simulink model "FinalSystem_WithRT"  (R2022b)
settings: Solver=FixedStepAuto  StartTime=0.0  StopTime=10.0  FixedStep=1e-3  RelTol=1e-3  EnableMultiTasking=on
undefined symbols (not defined in the file): D0, D1, D10, D11, D12, D13, D2, D3, D4, D5, D6, D7, D8, D9, PTA0, PTA1, PTA2, PTB23, PTB9, PTC16, PTC17, PTC2, PTC3, PTC4, PTD0, PTD1, PTD2, PTD3
libraries: frdmk64flib x17
settings Model: ExtModeTrigDuration=5  Creator=sarahalabdulrazzak  LastModifiedBy=TheCoaler
settings SolverCC: AlgebraicLoopSolver=TrustRegion
settings OptimizationCC: EnhancedBackFolding=on  PassReuseOutputArgsAs=Individual arguments  ZeroExternalMemoryAtStartup=off  ZeroInternalMemoryAtStartup=off  MaxStackSize=64  OptimizeBlockOrder=speed  DifferentSizesBufferReuse=on  OptimizationCustomize=off  EfficientTunableParamExpr=on
settings DebuggingCC: ParameterTunabilityLossMsg=error  UnconnectedInputMsg=warning  UnconnectedOutputMsg=warning  UnconnectedLineMsg=warning  SFMachineParentedDataDiag=warning
settings HardwareCC: ProdBitPerPointer=32  ProdBitPerSizeT=32  ProdBitPerPtrDiffT=32  ProdLargestAtomicInteger=Long  ProdLargestAtomicFloat=Double  ProdWordSize=32  ProdHWDeviceType=ARM Compatible->ARM Cortex
settings ModelReferenceCC: EnableRefExpFcnMdlSchedulingChecks=on
settings SFSimCC: MATLABDynamicMemAlloc=off
settings RTWCC: Description=Embedded Coder  SystemTargetFile=ert.tlc  HardwareBoard=NXP FRDM-K64F  TLCOptions="-aInlineSetEventsForThisBaseRateFcn=TLC_FALSE -aSuppressMultiTaskScheduler=TLC_FALSE  -aRateBasedStepFcn=0"  TemplateMakefile=ert_default_tmf  Toolchain=GNU Tools for ARM Embedded Processors
settings CodeAppCC: ForceParamTrailComments=on  IgnoreCustomStorageClasses=off  OperatorAnnotations=on  SimulinkDataObjDesc=on  SFDataObjDesc=on  InsertBlockDesc=on

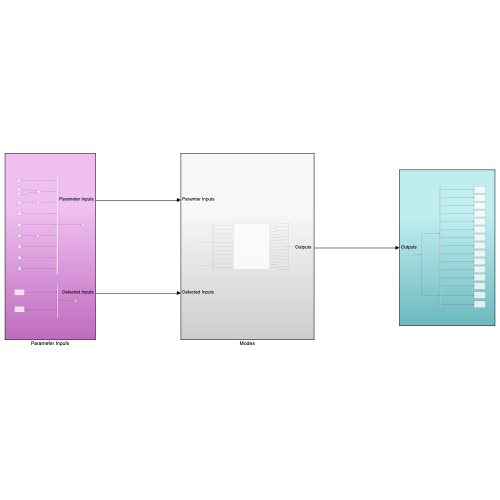
[thumbnail: Simulink's stored preview of the top-level diagram]
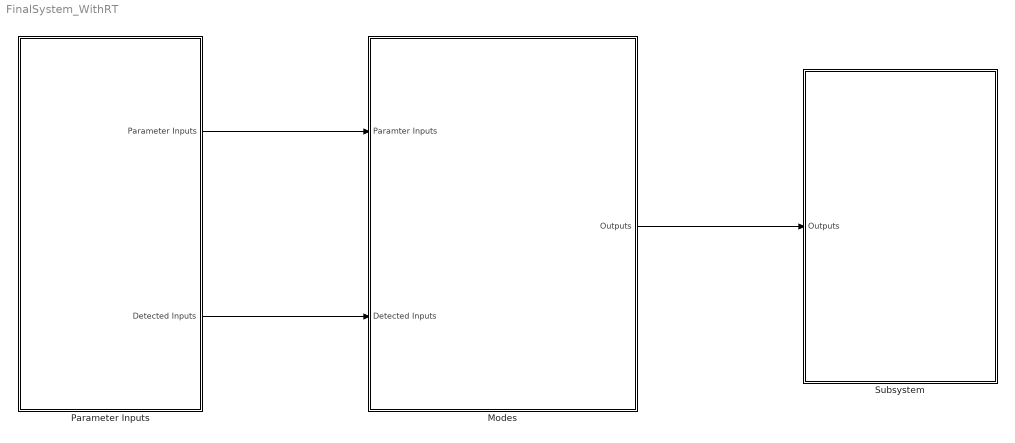
== system FinalSystem_WithRT ==
  Modes : Subsystem
  Parameter Inputs : Subsystem
  Subsystem : Subsystem
  wires:
  Parameter Inputs/1(Parameter Inputs) -> Modes/1(Paramter Inputs)
  Parameter Inputs/2(Detected Inputs) -> Modes/2(Detected Inputs)
  Modes/1("Outputs ") -> Subsystem/1("Outputs ")

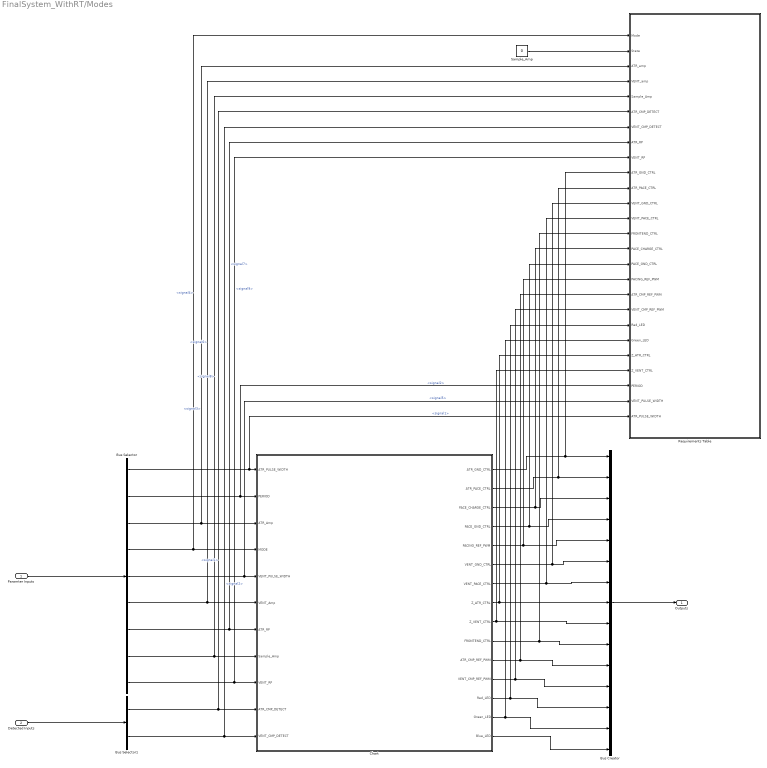
== system FinalSystem_WithRT/Modes ==
  Paramter Inputs : Inport
  Detected Inputs : Inport  Port=2
  Bus Creator : BusCreator  Inputs=15
  Bus Selector : BusSelector  OutputSignals=signal1,signal2,signal3,signal4,signal5,signal6,signal7,signal8,signal9
  Bus Selector1 : BusSelector  OutputSignals=signal1,signal2
  Chart : Stateflow chart  TreatAsAtomicUnit=on
  Requirements Table : Requirements Table  TreatAsAtomicUnit=on
  Sample_Amp : Constant  Value=0
  "Outputs " : Outport
  wires:
  Paramter Inputs/1 -> Bus Selector/1
  Detected Inputs/1 -> Bus Selector1/1
  Bus Selector/4 -> Requirements Table/1(Mode), Chart/4(MODE)  "<signal4>"
  Bus Selector/5 -> Requirements Table/25(VENT_PULSE_WIDTH), Chart/5(VENT_PULSE_WIDTH)  "<signal5>"
  Bus Selector/6 -> Requirements Table/4(VENT_amp), Chart/6(VENT_Amp)  "<signal6>"
  Bus Selector/7 -> Requirements Table/8(ATR_RP), Chart/7(ATR_RP)  "<signal7>"
  Bus Selector/8 -> Requirements Table/5(Sample_Amp), Chart/8(Sample_Amp)  "<signal8>"
  Bus Selector/9 -> Requirements Table/9(VENT_RP), Chart/9(VENT_RP)  "<signal9>"
  Bus Selector/1 -> Requirements Table/26(ATR_PULSE_WIDTH), Chart/1(ATR_PULSE_WIDTH)  "<signal1>"
  Bus Selector/2 -> Requirements Table/24(PERIOD), Chart/2(PERIOD)  "<signal2>"
  Bus Selector/3 -> Requirements Table/3(ATR_amp), Chart/3(ATR_Amp)  "<signal3>"
  Chart/1(ATR_GND_CTRL) -> Requirements Table/10(ATR_GND_CTRL), Bus Creator/1
  Chart/2(ATR_PACE_CTRL) -> Requirements Table/11(ATR_PACE_CTRL), Bus Creator/2
  Chart/3(PACE_CHARGE_CTRL) -> Requirements Table/15(PACE_CHARGE_CTRL), Bus Creator/3
  Chart/4(PACE_GND_CTRL) -> Requirements Table/16(PACE_GND_CTRL), Bus Creator/4
  Chart/5(PACING_REF_PWM) -> Requirements Table/17(PACING_REF_PWM), Bus Creator/5
  Chart/6(VENT_GND_CTRL) -> Requirements Table/12(VENT_GND_CTRL), Bus Creator/6
  Chart/7(VENT_PACE_CTRL) -> Requirements Table/13(VENT_PACE_CTRL), Bus Creator/7
  Chart/8(Z_ATR_CTRL) -> Requirements Table/22(Z_ATR_CTRL), Bus Creator/8
  Chart/9(Z_VENT_CTRL) -> Requirements Table/23(Z_VENT_CTRL), Bus Creator/9
  Chart/10(FRONTEND_CTRL) -> Requirements Table/14(FRONTEND_CTRL), Bus Creator/10
  Chart/11(ATR_CMP_REF_PWM) -> Requirements Table/18(ATR_CMP_REF_PWM), Bus Creator/11
  Chart/12(VENT_CMP_REF_PWM) -> Requirements Table/19(VENT_CMP_REF_PWM), Bus Creator/12
  Bus Creator/1 -> "Outputs "/1
  Chart/13(Red_LED) -> Requirements Table/20(Red_LED), Bus Creator/13
  Chart/14(Green_LED) -> Requirements Table/21(Green_LED), Bus Creator/14
  Chart/15(Blue_LED) -> Bus Creator/15
  Bus Selector1/1 -> Requirements Table/6(ATR_CMP_DETECT), Chart/10(ATR_CMP_DETECT)  "<signal1>"
  Bus Selector1/2 -> Requirements Table/7(VENT_CMP_DETECT), Chart/11(VENT_CMP_DETECT)  "<signal2>"
  Sample_Amp/1 -> Requirements Table/2(State)

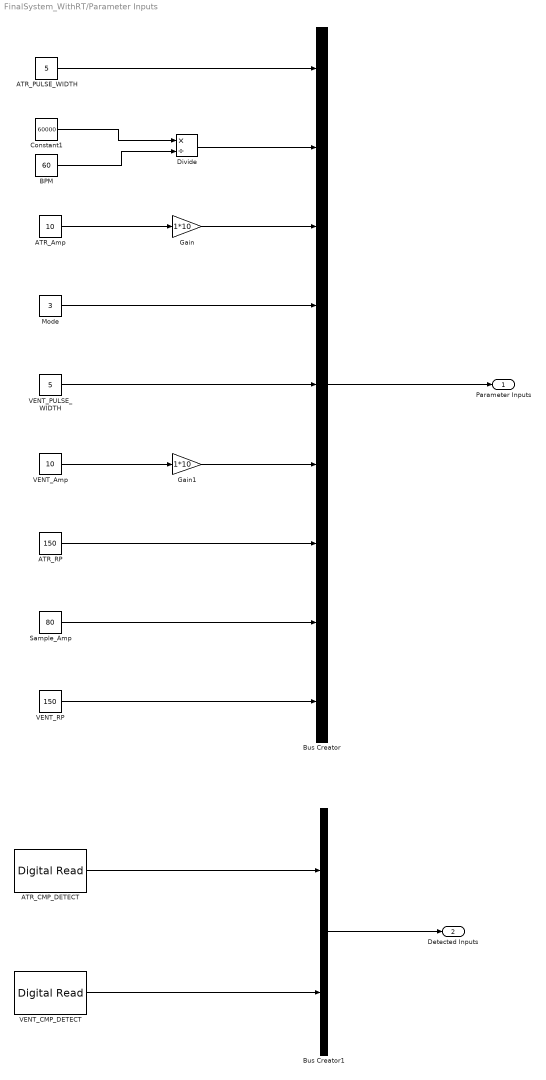
== system FinalSystem_WithRT/Parameter Inputs ==
  ATR_Amp : Constant  Value=10
  ATR_CMP_DETECT : frdmk64flib/Digital Read  Whichpin=PTC16 (D0)  SampleTime=-1
  ATR_PULSE_WIDTH : Constant  Value=5
  ATR_RP : Constant  Value=150
  BPM : Constant  Value=60
  Bus Creator : BusCreator  Inputs=9
  Bus Creator1 : BusCreator  Inputs=2
  Constant1 : Constant  Value=60000
  Divide : Product  Inputs=*/
  Gain : Gain  Gain=1*10
  Gain1 : Gain  Gain=1*10
  Mode : Constant  Value=3
  Sample_Amp : Constant  Value=80
  VENT_Amp : Constant  Value=10
  VENT_CMP_DETECT : frdmk64flib/Digital Read  Whichpin=PTC17 (D1)  SampleTime=-1
  VENT_PULSE_WIDTH : Constant  Value=5
  VENT_RP : Constant  Value=150
  Parameter Inputs : Outport
  Detected Inputs : Outport  Port=2
  wires:
  Bus Creator/1 -> Parameter Inputs/1
  ATR_PULSE_WIDTH/1 -> Bus Creator/1
  BPM/1 -> Divide/2
  Constant1/1 -> Divide/1
  Divide/1 -> Bus Creator/2
  ATR_Amp/1 -> Gain/1
  Gain/1 -> Bus Creator/3
  Mode/1 -> Bus Creator/4
  VENT_PULSE_WIDTH/1 -> Bus Creator/5
  VENT_Amp/1 -> Gain1/1
  Gain1/1 -> Bus Creator/6
  ATR_RP/1 -> Bus Creator/7
  Sample_Amp/1 -> Bus Creator/8
  VENT_RP/1 -> Bus Creator/9
  Bus Creator1/1 -> Detected Inputs/1
  VENT_CMP_DETECT/1 -> Bus Creator1/2
  ATR_CMP_DETECT/1 -> Bus Creator1/1

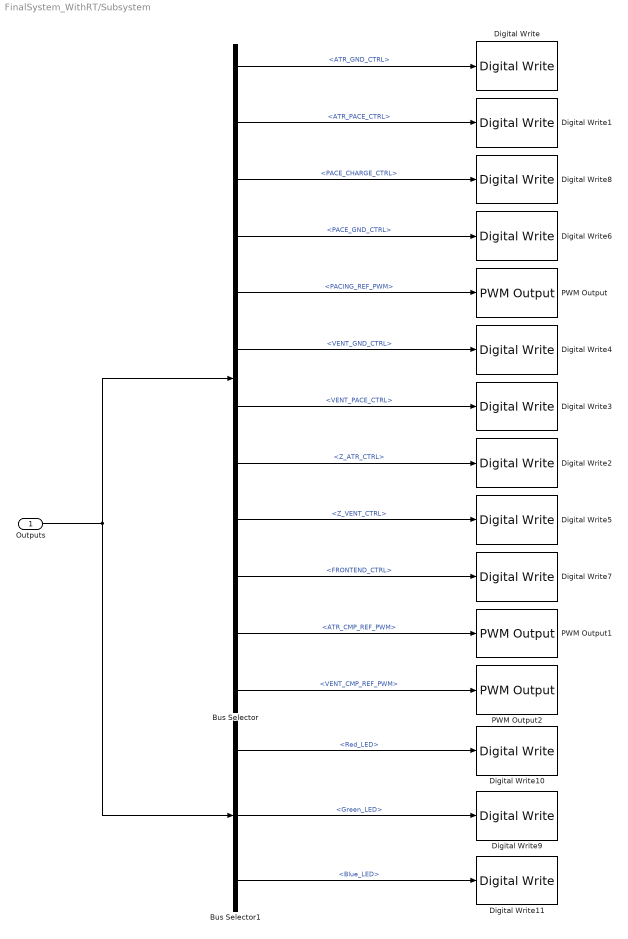
== system FinalSystem_WithRT/Subsystem ==
  "Outputs " : Inport
  Bus Selector : BusSelector  OutputSignals=ATR_GND_CTRL,ATR_PACE_CTRL,PACE_CHARGE_CTRL,PACE_GND_CTRL,PACING_REF_PWM,VENT_GND_CTRL,VENT_PACE_CTRL,Z_ATR_CTRL,Z_VENT_CTRL,FRONTEND_CTRL,ATR_CMP_REF_PWM,VENT_CMP_REF_PWM
  Bus Selector1 : BusSelector  OutputSignals=Red_LED,Green_LED,Blue_LED
  Digital Write : frdmk64flib/Digital Write  Whichpin=PTD2 (D11)
  Digital Write1 : frdmk64flib/Digital Write  Whichpin=PTA0 (D8)
  Digital Write10 : frdmk64flib/Digital Write  Whichpin=RED_LED
  Digital Write11 : frdmk64flib/Digital Write  Whichpin=BLUE_LED
  Digital Write2 : frdmk64flib/Digital Write  Whichpin=PTB23 (D4)
  Digital Write3 : frdmk64flib/Digital Write  Whichpin=PTC4 (D9)
  Digital Write4 : frdmk64flib/Digital Write  Whichpin=PTD3 (D12)
  Digital Write5 : frdmk64flib/Digital Write  Whichpin=PTC3 (D7)
  Digital Write6 : frdmk64flib/Digital Write  Whichpin=PTD0 (D10)
  Digital Write7 : frdmk64flib/Digital Write  Whichpin=PTD1 (D13)
  Digital Write8 : frdmk64flib/Digital Write  Whichpin=PTB9 (D2)
  Digital Write9 : frdmk64flib/Digital Write  Whichpin=GREEN_LED
  PWM Output : frdmk64flib/PWM Output  Whichpin=PTA2 (D5)  InitialFrequency=2000  InitialDutyCycle=0
  PWM Output1 : frdmk64flib/PWM Output  Whichpin=PTC2 (D6)  InitialFrequency=2000  InitialDutyCycle=0
  PWM Output2 : frdmk64flib/PWM Output  Whichpin=PTA1 (D3)  InitialFrequency=2000  InitialDutyCycle=0
  wires:
  Bus Selector/1 -> Digital Write/1  "<ATR_GND_CTRL>"
  Bus Selector/2 -> Digital Write1/1  "<ATR_PACE_CTRL>"
  Bus Selector/3 -> Digital Write8/1  "<PACE_CHARGE_CTRL>"
  Bus Selector/4 -> Digital Write6/1  "<PACE_GND_CTRL>"
  Bus Selector/5 -> PWM Output/1  "<PACING_REF_PWM>"
  Bus Selector/6 -> Digital Write4/1  "<VENT_GND_CTRL>"
  Bus Selector/7 -> Digital Write3/1  "<VENT_PACE_CTRL>"
  Bus Selector/8 -> Digital Write2/1  "<Z_ATR_CTRL>"
  Bus Selector/9 -> Digital Write5/1  "<Z_VENT_CTRL>"
  Bus Selector/10 -> Digital Write7/1  "<FRONTEND_CTRL>"
  Bus Selector/11 -> PWM Output1/1  "<ATR_CMP_REF_PWM>"
  Bus Selector/12 -> PWM Output2/1  "<VENT_CMP_REF_PWM>"
  "Outputs "/1 -> Bus Selector/1, Bus Selector1/1
  Bus Selector1/1 -> Digital Write10/1  "<Red_LED>"
  Bus Selector1/2 -> Digital Write9/1  "<Green_LED>"
  Bus Selector1/3 -> Digital Write11/1  "<Blue_LED>"

== stateflow chart FinalSystem_WithRT/Modes/Requirements Table ==
  (default) -> (junction 1073744062)
  (junction 1073744062) -> (junction 1073744063) : {
      | % SF_REQ_REV_07
      | }
  (junction 1073744063) -> (junction 1073744065) : {
      | % HEADER_ASSIGNMENTS
      |
      | }
  (junction 1073744065) -> (junction 1073744717) : {
      | % START_A_4
      | }
  (junction 1073744717) -> (junction 1073744719) : {
      | }
  (junction 1073744719) -> (junction 1073744721)
  (junction 1073744721) -> (junction 1073744723) [order 1] : [(0<Mode<5)]
  (junction 1073744721) -> (junction 1073744729) [order 2]
  (junction 1073744723) -> (junction 1073744725)
  (junction 1073744725) -> (junction 1073744727) : {
      | }
  (junction 1073744727) -> (junction 1073744729)
  (junction 1073744729) -> (junction 1073744731)
  (junction 1073744731) -> (junction 1073744733) : {
      | % END_A_4
      | }
  (junction 1073744733) -> (junction 1073744750) : {
      | % START_A_88
      | }
  (junction 1073744750) -> (junction 1073744752) : {
      | }
  (junction 1073744752) -> (junction 1073744754)
  (junction 1073744754) -> (junction 1073744756) [order 1] : [(-1<State<2)]
  (junction 1073744754) -> (junction 1073744762) [order 2]
  (junction 1073744756) -> (junction 1073744758)
  (junction 1073744758) -> (junction 1073744760) : {
      | }
  (junction 1073744760) -> (junction 1073744762)
  (junction 1073744762) -> (junction 1073744764)
  (junction 1073744764) -> (junction 1073744779) : {
      | % END_A_88
      | }
  (junction 1073744779) -> (junction 1073744783) : {
      | % START_A_94
      | }
  (junction 1073744783) -> (junction 1073744785) : {
      | }
  (junction 1073744785) -> (junction 1073744787)
  (junction 1073744787) -> (junction 1073744789) : {
      | }
  (junction 1073744789) -> (junction 1073744803) : {
      | % END_A_94
      | }
  (junction 1073744803) -> (junction 1073744077) : {
      | % START_R_1
      | }
  (junction 1073744077) -> (junction 1073744079) : {
      | }
  (junction 1073744079) -> (junction 1073744081)
  (junction 1073744081) -> (junction 1073744083) [order 1] : [((~((prev(PACE_CHARGE_CTRL)) == (0))))]
  (junction 1073744081) -> (junction 1073744089) [order 2]
  (junction 1073744083) -> (junction 1073744085) : {
      | reqtable_postcondition((((ATR_PACE_CTRL) == (0))) && (((VENT_PACE_CTRL) == (0))) && (((PACING_REF_PWM) >= (0) && (PACING_REF_PWM) <= (5))), 'R:1');
      |
      |
      | }
  (junction 1073744085) -> (junction 1073744087) : {
      | }
  (junction 1073744087) -> (junction 1073744089)
  (junction 1073744089) -> (junction 1073744091)
  (junction 1073744091) -> (junction 1073744093) : {
      | % END_R_1
      | }
  (junction 1073744093) -> (junction 1073744095) : {
      | % START_R_7
      | }
  (junction 1073744095) -> (junction 1073744097) : {
      | }
  (junction 1073744097) -> (junction 1073744099)
  (junction 1073744099) -> (junction 1073744101) [order 1] : [((~((prev(ATR_PACE_CTRL)) == (0)))) && ((~((prev(VENT_PACE_CTRL)) == (0))))]
  (junction 1073744099) -> (junction 1073744107) [order 2]
  (junction 1073744101) -> (junction 1073744103) : {
      | reqtable_postcondition((((PACE_CHARGE_CTRL) == (0))), 'R:2');
      |
      |
      | }
  (junction 1073744103) -> (junction 1073744105) : {
      | }
  (junction 1073744105) -> (junction 1073744107)
  (junction 1073744107) -> (junction 1073744109)
  (junction 1073744109) -> (junction 1073744111) : {
      | % END_R_7
      | }
  (junction 1073744111) -> (junction 1073744113) : {
      | % START_R_58
      | }
  (junction 1073744113) -> (junction 1073744115) : {
      | }
  (junction 1073744115) -> (junction 1073744117)
  (junction 1073744117) -> (junction 1073744119) [order 1] : [(((ATR_CMP_DETECT) == (1)))]
  (junction 1073744117) -> (junction 1073744125) [order 2]
  (junction 1073744119) -> (junction 1073744121) : {
      | reqtable_postcondition((((ATR_CMP_REF_PWM) > (5))), 'R:3');
      |
      |
      | }
  (junction 1073744121) -> (junction 1073744123) : {
      | }
  (junction 1073744123) -> (junction 1073744125)
  (junction 1073744125) -> (junction 1073744127)
  (junction 1073744127) -> (junction 1073744129) : {
      | % END_R_58
      | }
  (junction 1073744129) -> (junction 1073744131) : {
      | % START_R_64
      | }
  (junction 1073744131) -> (junction 1073744133) : {
      | }
  (junction 1073744133) -> (junction 1073744135)
  (junction 1073744135) -> (junction 1073744137) [order 1] : [(((ATR_CMP_DETECT) == (0)))]
  (junction 1073744135) -> (junction 1073744143) [order 2]
  (junction 1073744137) -> (junction 1073744139) : {
      | reqtable_postcondition((((ATR_CMP_REF_PWM) < (5))), 'R:4');
      |
      |
      | }
  (junction 1073744139) -> (junction 1073744141) : {
      | }
  (junction 1073744141) -> (junction 1073744143)
  (junction 1073744143) -> (junction 1073744145)
  (junction 1073744145) -> (junction 1073744147) : {
      | % END_R_64
      | }
  (junction 1073744147) -> (junction 1073744149) : {
      | % START_R_61
      | }
  (junction 1073744149) -> (junction 1073744151) : {
      | }
  (junction 1073744151) -> (junction 1073744153)
  (junction 1073744153) -> (junction 1073744155) [order 1] : [(((VENT_CMP_DETECT) == (1)))]
  (junction 1073744153) -> (junction 1073744161) [order 2]
  (junction 1073744155) -> (junction 1073744157) : {
      | reqtable_postcondition((((VENT_CMP_REF_PWM) > (5))), 'R:5');
      |
      |
      | }
  (junction 1073744157) -> (junction 1073744159) : {
      | }
  (junction 1073744159) -> (junction 1073744161)
  (junction 1073744161) -> (junction 1073744163)
  (junction 1073744163) -> (junction 1073744165) : {
      | % END_R_61
      | }
  (junction 1073744165) -> (junction 1073744167) : {
      | % START_R_67
      | }
  (junction 1073744167) -> (junction 1073744169) : {
      | }
  (junction 1073744169) -> (junction 1073744171)
  (junction 1073744171) -> (junction 1073744173) [order 1] : [(((VENT_CMP_DETECT) == (0)))]
  (junction 1073744171) -> (junction 1073744179) [order 2]
  (junction 1073744173) -> (junction 1073744175) : {
      | reqtable_postcondition((((VENT_CMP_REF_PWM) < (5))), 'R:6');
      |
      |
      | }
  (junction 1073744175) -> (junction 1073744177) : {
      | }
  (junction 1073744177) -> (junction 1073744179)
  (junction 1073744179) -> (junction 1073744181)
  (junction 1073744181) -> (junction 1073744183) : {
      | % END_R_67
      | }
  (junction 1073744183) -> (junction 1073744185) : {
      | % START_R_46
      | }
  (junction 1073744185) -> (junction 1073744187) : {
      | }
  (junction 1073744187) -> (junction 1073744189) : {
      |
      |
      | }
  (junction 1073744189) -> (junction 1073744191) : {
      | }
  (junction 1073744191) -> (junction 1073744193) : {
      | % START_R_52
      | }
  (junction 1073744193) -> (junction 1073744195) : {
      | }
  (junction 1073744195) -> (junction 1073744197)
  (junction 1073744197) -> (junction 1073744199) [order 1] : [(((Mode) == (1))) && (((State) == (1)))]
  (junction 1073744197) -> (junction 1073744205) [order 2]
  (junction 1073744199) -> (junction 1073744201) : {
      | reqtable_postcondition((((ATR_PACE_CTRL) == (0))) && (((VENT_PACE_CTRL) == (0))) && (((PACE_GND_CTRL) == (1))) && (((Z_ATR_CTRL) == (0))) && (((Z_VENT_CTRL) == (0))) && (((ATR_GND_CTRL) == (1))) && (((VENT_GND_CTRL) == (0))) && (((Red_LED) == (0))) && (((Green_LED) == (0))) && (((PACING_REF_PWM) == (ATR_amp))) && (((PACE_CHARGE_CTRL) == (1))) && (((FRONTEND_CTRL) == (0))), 'R:7.1');
      |
      |
      | }
  (junction 1073744201) -> (junction 1073744203) : {
      | }
  (junction 1073744203) -> (junction 1073744205)
  (junction 1073744205) -> (junction 1073744207)
  (junction 1073744207) -> (junction 1073744209) : {
      | % END_R_52
      | }
  (junction 1073744209) -> (junction 1073744211) : {
      | % START_R_55
      | }
  (junction 1073744211) -> (junction 1073744213) : {
      | }
  (junction 1073744213) -> (junction 1073744215)
  (junction 1073744215) -> (junction 1073744217) [order 1] : [(((Mode) == (1))) && (((State) == (0)))]
  (junction 1073744215) -> (junction 1073744223) [order 2]
  (junction 1073744217) -> (junction 1073744219) : {
      | reqtable_postcondition((((ATR_PACE_CTRL) == (1))) && (((VENT_PACE_CTRL) == (0))) && (((PACE_GND_CTRL) == (1))) && (((Z_ATR_CTRL) == (0))) && (((Z_VENT_CTRL) == (0))) && (((ATR_GND_CTRL) == (0))) && (((VENT_GND_CTRL) == (0))) && (((Red_LED) == (1))) && (((Green_LED) == (0))) && (((PACING_REF_PWM) == (ATR_amp))) && (((PACE_CHARGE_CTRL) == (0))) && (((FRONTEND_CTRL) == (0))), 'R:7.2');
      |
      |
      | }
  (junction 1073744219) -> (junction 1073744221) : {
      | }
  (junction 1073744221) -> (junction 1073744223)
  (junction 1073744223) -> (junction 1073744225)
  (junction 1073744225) -> (junction 1073744227) : {
      | % END_R_55
      | }
  (junction 1073744227) -> (junction 1073744229) : {
      | % END_R_46
      | }
  (junction 1073744229) -> (junction 1073744339) : {
      | % START_R_49
      | }
  (junction 1073744339) -> (junction 1073744341) : {
      | }
  (junction 1073744341) -> (junction 1073744343) : {
      |
      |
      | }
  (junction 1073744343) -> (junction 1073744345) : {
      | }
  (junction 1073744345) -> (junction 1073744441) : {
      | % START_R_76
      | }
  (junction 1073744441) -> (junction 1073744443) : {
      | }
  (junction 1073744443) -> (junction 1073744445)
  (junction 1073744445) -> (junction 1073744447) [order 1] : [(((Mode) == (3))) && (((State) == (1)))]
  (junction 1073744445) -> (junction 1073744453) [order 2]
  (junction 1073744447) -> (junction 1073744449) : {
      | reqtable_postcondition((((ATR_PACE_CTRL) == (0))) && (((VENT_PACE_CTRL) == (0))) && (((PACE_GND_CTRL) == (1))) && (((Z_ATR_CTRL) == (0))) && (((Z_VENT_CTRL) == (0))) && (((ATR_GND_CTRL) == (0))) && (((VENT_GND_CTRL) == (1))) && (((Red_LED) == (0))) && (((Green_LED) == (0))) && (((PACING_REF_PWM) == (VENT_amp))) && (((PACE_CHARGE_CTRL) == (1))) && (((FRONTEND_CTRL) == (0))), 'R:8.1');
      |
      |
      | }
  (junction 1073744449) -> (junction 1073744451) : {
      | }
  (junction 1073744451) -> (junction 1073744453)
  (junction 1073744453) -> (junction 1073744455)
  (junction 1073744455) -> (junction 1073744457) : {
      | % END_R_76
      | }
  (junction 1073744457) -> (junction 1073744462) : {
      | % START_R_79
      | }
  (junction 1073744462) -> (junction 1073744464) : {
      | }
  (junction 1073744464) -> (junction 1073744466)
  (junction 1073744466) -> (junction 1073744468) [order 1] : [(((Mode) == (3))) && (((State) == (0)))]
  (junction 1073744466) -> (junction 1073744474) [order 2]
  (junction 1073744468) -> (junction 1073744470) : {
      | reqtable_postcondition((((ATR_PACE_CTRL) == (0))) && (((VENT_PACE_CTRL) == (1))) && (((PACE_GND_CTRL) == (1))) && (((Z_ATR_CTRL) == (0))) && (((Z_VENT_CTRL) == (0))) && (((ATR_GND_CTRL) == (0))) && (((VENT_GND_CTRL) == (0))) && (((Red_LED) == (1))) && (((Green_LED) == (0))) && (((PACING_REF_PWM) == (VENT_amp))) && (((PACE_CHARGE_CTRL) == (0))) && (((FRONTEND_CTRL) == (0))), 'R:8.2');
      |
      |
      | }
  (junction 1073744470) -> (junction 1073744472) : {
      | }
  (junction 1073744472) -> (junction 1073744474)
  (junction 1073744474) -> (junction 1073744476)
  (junction 1073744476) -> (junction 1073744478) : {
      | % END_R_79
      | }
  (junction 1073744478) -> (junction 1073744357) : {
      | % END_R_49
      | }
  (junction 1073744357) -> (junction 1073744271) : {
      | % START_R_10
      | }
  (junction 1073744271) -> (junction 1073744273) : {
      | }
  (junction 1073744273) -> (junction 1073744275) : {
      |
      |
      | }
  (junction 1073744275) -> (junction 1073744277) : {
      | }
  (junction 1073744277) -> (junction 1073744483) : {
      | % START_R_70
      | }
  (junction 1073744483) -> (junction 1073744485) : {
      | }
  (junction 1073744485) -> (junction 1073744487)
  (junction 1073744487) -> (junction 1073744489) [order 1] : [(((Mode) == (2))) && (((State) == (1)))]
  (junction 1073744487) -> (junction 1073744495) [order 2]
  (junction 1073744489) -> (junction 1073744491) : {
      | reqtable_postcondition((((ATR_PACE_CTRL) == (0))) && (((VENT_PACE_CTRL) == (0))) && (((PACE_GND_CTRL) == (1))) && (((Z_ATR_CTRL) == (0))) && (((Z_VENT_CTRL) == (0))) && (((ATR_GND_CTRL) == (1))) && (((VENT_GND_CTRL) == (0))) && (((Red_LED) == (0))) && (((Green_LED) == (1))) && (((PACING_REF_PWM) == (ATR_amp))) && (((PACE_CHARGE_CTRL) == (1))) && (((ATR_CMP_REF_PWM) == (Sample_Amp))) && (((FRONTEND_CTRL) == (1))), 'R:9.1');
      |
      |
      | }
  (junction 1073744491) -> (junction 1073744493) : {
      | }
  (junction 1073744493) -> (junction 1073744495)
  (junction 1073744495) -> (junction 1073744497)
  (junction 1073744497) -> (junction 1073744499) : {
      | % END_R_70
      | }
  (junction 1073744499) -> (junction 1073744504) : {
      | % START_R_73
      | }
  (junction 1073744504) -> (junction 1073744506) : {
      | }
  (junction 1073744506) -> (junction 1073744508)
  (junction 1073744508) -> (junction 1073744510) [order 1] : [(((Mode) == (2))) && (((State) == (0)))]
  (junction 1073744508) -> (junction 1073744516) [order 2]
  (junction 1073744510) -> (junction 1073744512) : {
      | reqtable_postcondition((((ATR_PACE_CTRL) == (1))) && (((VENT_PACE_CTRL) == (0))) && (((PACE_GND_CTRL) == (1))) && (((Z_ATR_CTRL) == (0))) && (((Z_VENT_CTRL) == (0))) && (((ATR_GND_CTRL) == (0))) && (((VENT_GND_CTRL) == (0))) && (((Red_LED) == (1))) && (((Green_LED) == (0))) && (((PACING_REF_PWM) == (ATR_amp))) && (((PACE_CHARGE_CTRL) == (0))) && (((FRONTEND_CTRL) == (0))), 'R:9.2');
      |
      |
      | }
  (junction 1073744512) -> (junction 1073744514) : {
      | }
  (junction 1073744514) -> (junction 1073744516)
  (junction 1073744516) -> (junction 1073744518)
  (junction 1073744518) -> (junction 1073744520) : {
      | % END_R_73
      | }
  (junction 1073744520) -> (junction 1073744289) : {
      | % END_R_10
      | }
  (junction 1073744289) -> (junction 1073744407) : {
      | % START_R_13
      | }
  (junction 1073744407) -> (junction 1073744409) : {
      | }
  (junction 1073744409) -> (junction 1073744411) : {
      |
      |
      | }
  (junction 1073744411) -> (junction 1073744413) : {
      | }
  (junction 1073744413) -> (junction 1073744525) : {
      | % START_R_82
      | }
  (junction 1073744525) -> (junction 1073744527) : {
      | }
  (junction 1073744527) -> (junction 1073744529)
  (junction 1073744529) -> (junction 1073744531) [order 1] : [(((Mode) == (4))) && (((State) == (1)))]
  (junction 1073744529) -> (junction 1073744537) [order 2]
  (junction 1073744531) -> (junction 1073744533) : {
      | reqtable_postcondition((((ATR_PACE_CTRL) == (0))) && (((VENT_PACE_CTRL) == (0))) && (((PACE_GND_CTRL) == (1))) && (((Z_ATR_CTRL) == (0))) && (((Z_VENT_CTRL) == (0))) && (((ATR_GND_CTRL) == (0))) && (((VENT_GND_CTRL) == (1))) && (((Red_LED) == (0))) && (((Green_LED) == (1))) && (((PACING_REF_PWM) == (VENT_amp))) && (((PACE_CHARGE_CTRL) == (1))) && (((ATR_CMP_REF_PWM) == (Sample_Amp))) && (((FRONTEND_CTRL) == (1))), 'R:10.1');
      |
      |
      | }
  (junction 1073744533) -> (junction 1073744535) : {
      | }
  (junction 1073744535) -> (junction 1073744537)
  (junction 1073744537) -> (junction 1073744539)
  (junction 1073744539) -> (junction 1073744541) : {
      | % END_R_82
      | }
  (junction 1073744541) -> (junction 1073744546) : {
      | % START_R_85
      | }
  (junction 1073744546) -> (junction 1073744548) : {
      | }
  (junction 1073744548) -> (junction 1073744550)
  (junction 1073744550) -> (junction 1073744552) [order 1] : [(((Mode) == (4))) && (((State) == (0)))]
  (junction 1073744550) -> (junction 1073744558) [order 2]
  (junction 1073744552) -> (junction 1073744554) : {
      | reqtable_postcondition((((ATR_PACE_CTRL) == (0))) && (((VENT_PACE_CTRL) == (1))) && (((PACE_GND_CTRL) == (1))) && (((Z_ATR_CTRL) == (0))) && (((Z_VENT_CTRL) == (0))) && (((ATR_GND_CTRL) == (0))) && (((VENT_GND_CTRL) == (0))) && (((Red_LED) == (1))) && (((Green_LED) == (0))) && (((PACING_REF_PWM) == (VENT_amp))) && (((PACE_CHARGE_CTRL) == (0))) && (((FRONTEND_CTRL) == (0))), 'R:10.2');
      |
      |
      | }
  (junction 1073744554) -> (junction 1073744556) : {
      | }
  (junction 1073744556) -> (junction 1073744558)
  (junction 1073744558) -> (junction 1073744560)
  (junction 1073744560) -> (junction 1073744562) : {
      | % END_R_85
      | }
  (junction 1073744562) -> (junction 1073744425) : {
      | % END_R_13
      | }
  data: Mode input; State input; ATR_amp input; VENT_amp input; Sample_Amp input; ATR_CMP_DETECT input; VENT_CMP_DETECT input; ATR_RP input; VENT_RP input; ATR_GND_CTRL input; ATR_PACE_CTRL input; VENT_GND_CTRL input; VENT_PACE_CTRL input; FRONTEND_CTRL input; PACE_CHARGE_CTRL input; PACE_GND_CTRL input; PACING_REF_PWM input; ATR_CMP_REF_PWM input; VENT_CMP_REF_PWM input; Red_LED input; Green_LED input; Z_ATR_CTRL input; Z_VENT_CTRL input; PERIOD input; VENT_PULSE_WIDTH input; ATR_PULSE_WIDTH input

== stateflow chart FinalSystem_WithRT/Modes/Chart ==
  state AOO
    entry:
    %Charge primary capcitor C22
    ATR_PACE_CTRL=LOW
    VENT_PACE_CTRL=LOW
    PACING_REF_PWM = ATR_Amp
    PACE_CHARGE_CTRL = HIGH
    %Discharge block capacitor C21
    PACE_GND_CTRL = HIGH
    %VENT_PACE_CTRL = LOW
    Z_ATR_CTRL = LOW
    Z_VENT_CTRL = LOW
    %ATR_PACE_CTRL = LOW
    ATR_GND_CTRL = HIGH
    VENT_GND_CTRL = LOW
    %use LED  to verify state
    Red_LED=false
    Green_LED=false
    Blue_LED=false
  state Identify_Mode_Path
    entry:
    % MODE = 1 (AOO)
    % MODE = 2 (AAI)
    % MODE = 3 (VOO)
    % MODE = 4 (VVI)
    %
    %pacemaker disconnected
    %stop sensing
    PACE_CHARGE_CTRL = LOW
    VENT_PACE_CTRL = LOW
    ATR_PACE_CTRL = LOW
    PACE_GND_CTRL = LOW
    ATR_GND_CTRL = LOW
    VENT_GND_CTRL = LOW
    Z_ATR_CTRL = LOW
    Z_VENT_CTRL = LOW
    FRONTEND_CTRL = LOW
  state AOO_ATR_PULSE
    entry:
    %Discharge C22 primary capacitor
    %Charge C21 block capacitor
    PACE_CHARGE_CTRL = LOW
    PACE_GND_CTRL = HIGH
    ATR_PACE_CTRL = HIGH
    ATR_GND_CTRL = LOW
    Z_ATR_CTRL = LOW
    Z_VENT_CTRL = LOW
    VENT_GND_CTRL = LOW
    VENT_PACE_CTRL  = LOW
    PACING_REF_PWM = ATR_Amp
    %use LED  to verify state
    Red_LED=true
    Green_LED=false
    Blue_LED=false
  state AAI
    entry:
    %sensing ON
    FRONTEND_CTRL = HIGH
    %Charge primary capcitor C22
    ATR_PACE_CTRL=LOW
    VENT_PACE_CTRL=LOW
    PACING_REF_PWM = ATR_Amp
    PACE_CHARGE_CTRL = HIGH
    %Discharge block capacitor C21
    PACE_GND_CTRL = HIGH
    VENT_PACE_CTRL = LOW
    Z_ATR_CTRL = LOW
    Z_VENT_CTRL = LOW
    ATR_GND_CTRL = HIGH
    VENT_GND_CTRL = LOW
    ATR_CMP_REF_PWM = Sample_Amp
    %use LED  to verify state
    Red_LED=false
    Blue_LED=false
    Green_LED=false
  state AAI_ATR_PULSE
    entry:
    %sensing OFF
    FRONTEND_CTRL = LOW
    %Discharge C22 primary capacitor
    %Charge C21 block capacitor
    PACE_CHARGE_CTRL = LOW
    PACE_GND_CTRL = HIGH
    ATR_PACE_CTRL = HIGH
    ATR_GND_CTRL = LOW
    Z_ATR_CTRL = LOW
    Z_VENT_CTRL = LOW
    VENT_GND_CTRL = LOW
    VENT_PACE_CTRL  = LOW
    PACING_REF_PWM = ATR_Amp
    %use LED  to verify state
    Red_LED=false
    Green_LED=false
    Blue_LED=true
  state VOO
    entry:
    %Charge primary capcitor C22
    ATR_PACE_CTRL=LOW
    VENT_PACE_CTRL=LOW
    PACING_REF_PWM = VENT_Amp
    PACE_CHARGE_CTRL = HIGH
    %Discharge block capacitor C21
    PACE_GND_CTRL = HIGH
    %VENT_PACE_CTRL = LOW
    Z_ATR_CTRL = LOW
    Z_VENT_CTRL = LOW
    %ATR_PACE_CTRL = LOW
    ATR_GND_CTRL = LOW
    VENT_GND_CTRL = HIGH
    %use LED  to verify state
    Red_LED=false
    Green_LED=false
    Blue_LED=false
  state VOO_VENT_PULSE
    entry:
    %Discharge C22 primary capacitor
    %Charge C21 block capacitor
    PACE_CHARGE_CTRL = LOW
    PACE_GND_CTRL = HIGH
    ATR_PACE_CTRL = LOW
    ATR_GND_CTRL = LOW
    Z_ATR_CTRL = LOW
    Z_VENT_CTRL = LOW
    VENT_GND_CTRL = LOW
    VENT_PACE_CTRL  = HIGH
    PACING_REF_PWM = VENT_Amp
    %use LED  to verify state
    Red_LED=false
    Green_LED=true
    Blue_LED=false
  state VVI
    entry:
    %sensing ON
    FRONTEND_CTRL = HIGH
    %Charge primary capcitor C22
    ATR_PACE_CTRL=LOW
    VENT_PACE_CTRL= LOW
    PACING_REF_PWM = VENT_Amp
    PACE_CHARGE_CTRL = HIGH
    %Discharge block capacitor C21
    PACE_GND_CTRL = HIGH
    VENT_PACE_CTRL = LOW
    Z_ATR_CTRL = LOW
    Z_VENT_CTRL = LOW
    ATR_GND_CTRL = LOW
    VENT_GND_CTRL = HIGH
    VENT_CMP_REF_PWM = Sample_Amp
    %use LED  to verify state
    Red_LED=true
    Green_LED=false
    Blue_LED=false
  state VVI_VENT_PULSE
    %sensing OFF
    FRONTEND_CTRL = LOW
    %Discharge C22 primary capacitor
    %Charge C21 block capacitor
    PACE_CHARGE_CTRL = LOW
    PACE_GND_CTRL = HIGH
    ATR_PACE_CTRL = LOW
    ATR_GND_CTRL = LOW
    Z_ATR_CTRL = LOW
    Z_VENT_CTRL = LOW
    VENT_GND_CTRL = LOW
    VENT_PACE_CTRL  = HIGH
    PACING_REF_PWM = VENT_Amp
    %use LED  to verify state
    Red_LED=false
    Green_LED=true
    Blue_LED=false
  (default) -> Identify_Mode_Path
  AOO -> AOO_ATR_PULSE : after(PERIOD - ATR_PULSE_WIDTH,msec)
  Identify_Mode_Path -> AOO [order 1] : [MODE == 1]
  AOO_ATR_PULSE -> AOO : after(ATR_PULSE_WIDTH,msec)
  AAI_ATR_PULSE -> AAI : after(ATR_PULSE_WIDTH,msec)
  Identify_Mode_Path -> AAI [order 2] : [MODE == 2]
  AAI -> (junction 41)
  (junction 41) -> AAI_ATR_PULSE [order 1] : after(PERIOD - ATR_PULSE_WIDTH,msec)[ATR_CMP_DETECT == LOW]
  (junction 41) -> (junction 35) [order 2] : [ATR_CMP_DETECT == HIGH]
  (junction 35) -> AAI : after(ATR_RP, msec)
  VOO -> VOO_VENT_PULSE : after(PERIOD - VENT_PULSE_WIDTH,msec)
  Identify_Mode_Path -> VOO [order 3] : [MODE == 3]
  VOO_VENT_PULSE -> VOO : after(VENT_PULSE_WIDTH,msec)
  VVI_VENT_PULSE -> VVI : after(VENT_PULSE_WIDTH,msec)
  Identify_Mode_Path -> VVI [order 4] : [MODE == 4]
  VVI -> (junction 61)
  (junction 61) -> VVI_VENT_PULSE [order 1] : after(PERIOD - VENT_PULSE_WIDTH,msec)[VENT_CMP_DETECT == LOW]
  (junction 61) -> (junction 59) [order 2] : [VENT_CMP_DETECT == HIGH]
  (junction 59) -> VVI : after(VENT_RP, msec)
  data: ATR_PULSE_WIDTH input; PERIOD input; ATR_Amp input; MODE input; VENT_PULSE_WIDTH input; VENT_Amp input; ATR_RP input; Sample_Amp input; VENT_RP input; ATR_CMP_DETECT input; VENT_CMP_DETECT input; HIGH local =1; LOW local =0; ATR_GND_CTRL output; ATR_PACE_CTRL output; PACE_CHARGE_CTRL output; PACE_GND_CTRL output; PACING_REF_PWM output; VENT_GND_CTRL output; VENT_PACE_CTRL output; Z_ATR_CTRL output; Z_VENT_CTRL output; FRONTEND_CTRL output; ATR_CMP_REF_PWM output; VENT_CMP_REF_PWM output; Red_LED output; Green_LED output; Blue_LED output
